simulink model "cartesianRelativeStatePropagator"  (R2023a)
settings: Solver=ode4  StartTime=0.0  StopTime=10.0  FixedStep=dt  RelTol=1e-3
settings Model: Creator=ndelurgio  LastModifiedBy=ndelurgio

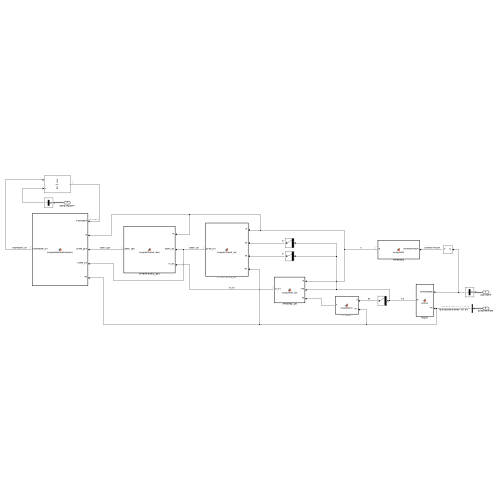
[thumbnail: Simulink's stored preview of the top-level diagram]
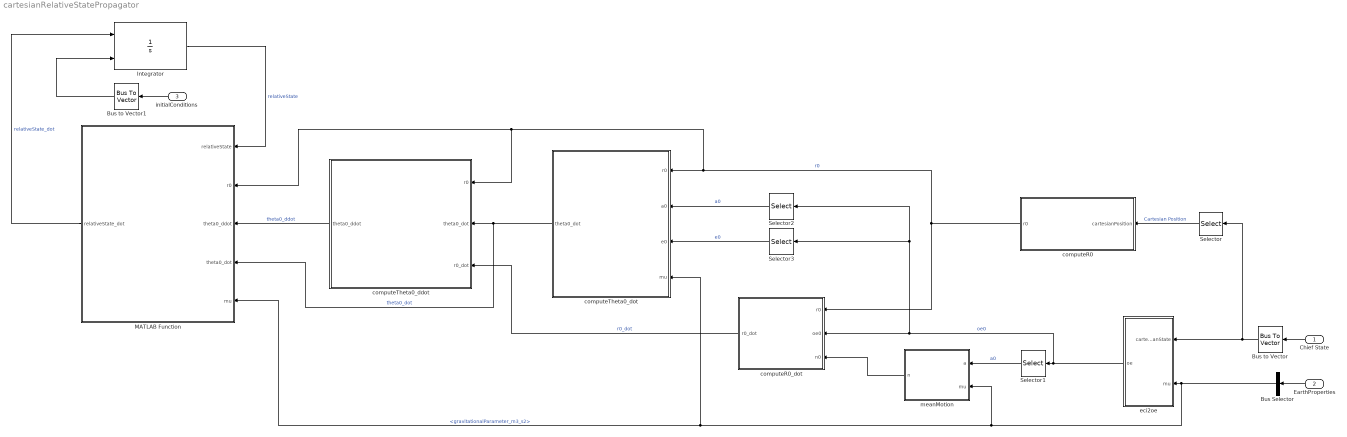
== system cartesianRelativeStatePropagator ==
  Chief State : Inport  OutDataTypeStr=Bus: cartesianState
  EarthProperties : Inport  Port=2  OutDataTypeStr=Bus: earthProperties
  initialConditions : Inport  Port=3  OutDataTypeStr=Bus: relativeCartesianState
  Bus Selector : BusSelector  OutputSignals=gravitationalParameter_m3_s2
  Bus to Vector : BusToVector
  Bus to Vector1 : BusToVector
  Integrator : Integrator  InitialConditionSource=external
  MATLAB Function : MATLAB Function  TreatAsAtomicUnit=on
  Selector : Selector  InputPortWidth=6  IndexOptions=Index vector (dialog)  Indices=1:3  OutputSizes=1
  Selector1 : Selector  InputPortWidth=6  IndexOptions=Index vector (dialog)  Indices=1  OutputSizes=1
  Selector2 : Selector  InputPortWidth=6  IndexOptions=Index vector (dialog)  Indices=1  OutputSizes=1
  Selector3 : Selector  InputPortWidth=6  IndexOptions=Index vector (dialog)  Indices=2  OutputSizes=1
  computeR0 : MATLAB Function  TreatAsAtomicUnit=on
  computeR0_dot : MATLAB Function  TreatAsAtomicUnit=on
  computeTheta0_ddot : MATLAB Function  TreatAsAtomicUnit=on
  computeTheta0_dot : MATLAB Function  TreatAsAtomicUnit=on
  eci2oe : MATLAB Function  TreatAsAtomicUnit=on
  meanMotion : MATLAB Function  TreatAsAtomicUnit=on
  wires:
  eci2oe/1(oe) -> Selector3/1, Selector2/1, computeR0_dot/2(oe0), Selector1/1  "oe0"
  EarthProperties/1 -> Bus Selector/1
  Bus Selector/1 -> meanMotion/2(mu), MATLAB Function/5(mu), computeTheta0_dot/4(mu), eci2oe/2(mu)  "<gravitationalParameter_m3_s2>"
  Selector/1 -> computeR0/1(cartesianPosition)  "Cartesian Position"
  Selector1/1 -> meanMotion/1(a)  "a0"
  meanMotion/1(n) -> computeR0_dot/3(n0)
  computeR0/1(r0) -> MATLAB Function/2(r0), computeTheta0_ddot/1(r0), computeTheta0_dot/1(r0), computeR0_dot/1(r0)  "r0"
  Selector2/1 -> computeTheta0_dot/2(a0)  "a0"
  Selector3/1 -> computeTheta0_dot/3(e0)  "e0"
  computeTheta0_dot/1(theta0_dot) -> MATLAB Function/4(theta0_dot), computeTheta0_ddot/2(theta0_dot)  "theta0_dot"
  computeR0_dot/1(r0_dot) -> computeTheta0_ddot/3(r0_dot)  "r0_dot"
  Integrator/1 -> MATLAB Function/1(relativeState)  "relativeState"
  MATLAB Function/1(relativeState_dot) -> Integrator/1  "relativeState_dot"
  computeTheta0_ddot/1(theta0_ddot) -> MATLAB Function/3(theta0_ddot)  "theta0_ddot"
  initialConditions/1 -> Bus to Vector1/1
  Bus to Vector1/1 -> Integrator/2
  Chief State/1 -> Bus to Vector/1
  Bus to Vector/1 -> Selector/1, eci2oe/1(cartesianState)

== matlab function cartesianRelativeStatePropagator/computeR0 ==
  data: cartesianPosition input; r0 output
function r0  = computeR0(cartesianPosition)
r0 = computeR0(cartesianPosition);
end

== matlab function cartesianRelativeStatePropagator/eci2oe ==
  data: cartesianState input; oe output; mu input
function oe = eci2oe(cartesianState,mu)
[oe,~,~,~] = eci2oe( cartesianState , mu );
end

== matlab function cartesianRelativeStatePropagator/meanMotion ==
  data: a input; mu input; n output
function n  = meanMotion(a,mu)
n = meanMotion(mu,a);
end

== matlab function cartesianRelativeStatePropagator/computeR0_dot ==
  data: r0 input; oe0 input; r0_dot output; n0 input
function r0_dot  = computeR0_dot(r0,oe0, n0)
r0_dot = computeR0_dot(oe0, n0, r0);
end

== matlab function cartesianRelativeStatePropagator/computeTheta0_dot ==
  data: r0 input; a0 input; e0 input; theta0_dot output; mu input
function theta0_dot = computeTheta0_dot(r0,a0,e0,mu)
theta0_dot = computeTheta0_dot(r0,mu,a0,e0);
end

== matlab function cartesianRelativeStatePropagator/computeTheta0_ddot ==
  data: r0 input; theta0_dot input; theta0_ddot output; r0_dot input
function theta0_ddot = computeTheta0_ddot(r0,theta0_dot,r0_dot)
theta0_ddot = computeTheta0_ddot(r0,r0_dot,theta0_dot);
end

== matlab function cartesianRelativeStatePropagator/MATLAB Function ==
  data: relativeState input; relativeState_dot output; r0 input; theta0_ddot input; theta0_dot input; mu input
function relativeState_dot = computeRelativeDynamics(relativeState,r0,theta0_ddot,theta0_dot,mu)
relativeState_dot = computeRelativeDynamics(relativeState,r0,theta0_dot,theta0_ddot,mu);
end
